simulink model "ThirdCOMController"  (Simulink 7.9)
settings: Solver=ode3  StartTime=0.0  StopTime=inf  RelTol=1e-3
libraries: dspmtrx3 x5, simulink x2, simulink_extras x1, utility x1
settings Model: Creator=jorhabib  LastModifiedBy=jorhabib

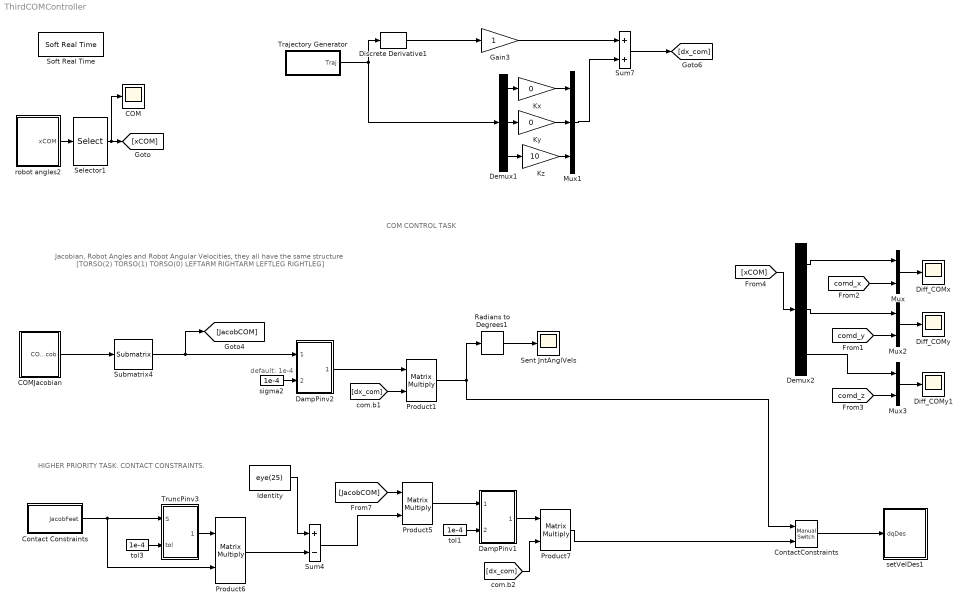
== system ThirdCOMController ==
  note: COM CONTROL TASK
  note: default: 1e-4
  note: Jacobian, Robot Angles and Robot Angular Velocities, they all have the same structure
      | [TORSO(2)  TORSO(1)  TORSO(0)    LEFTARM    RIGHTARM    LEFTLEG    RIGHTLEG]
  note: HIGHER PRIORITY TASK. CONTACT CONSTRAINTS.
  COM : Scope
      settings: TimeRange=100  YMin=-0.1  YMax=0.175
  COMJacobian : Subsystem
  Contact Constraints : Subsystem
  ContactConstraints : simulink/Signal Routing/Manual Switch  sw=1  action=0  varsize=off
  DampPinv1 : Subsystem  mask{tol=1e-4}
      mask prompts: tol "Tolerance"
  DampPinv2 : Subsystem  mask{tol=1e-4}
      mask prompts: tol "Tolerance"
  Demux1 : Demux  Outputs=3
  Demux2 : Demux  Outputs=3
  Diff_COMx : Scope
      settings: TimeRange=100  YMin=0.018  YMax=0.033  SaveName=ScopeData2
  Diff_COMy : Scope
      settings: TimeRange=100  YMin=-0.075  YMax=-0.062  SaveName=ScopeData5
  Diff_COMy1 : Scope
      settings: TimeRange=100  YMin=0.49  YMax=0.55  SaveName=ScopeData3
  Discrete Derivative1 : simulink/Discrete/Discrete Derivative  gainval=1.0  ICPrevScaledInput=0.0  InputProcessing=Inherited  OutMin=[]  OutMax=[]  OutDataType=fixdt(1, 16)  OutScaling=2^-10  DoSatur=off
  Gain3 : Gain
  Identity : Constant  Value=eye(25)
  Kx : Gain  Gain=0
  Ky : Gain  Gain=0
  Kz : Gain  Gain=10
  Mux : Mux  Inputs=2
  Mux1 : Mux  Inputs=3
  Mux2 : Mux  Inputs=2
  Mux3 : Mux  Inputs=2
  Product{1,5..7} (4 alike) : Product  Multiplication=Matrix(*)  RndMeth=Zero
  Radians to Degrees1 : simulink_extras/Transformations/Radians to Degrees
  Selector1 : Selector  IndexMode=Zero-based  InputPortWidth=7  IndexOptions=Index vector (dialog)  Indices=[0:2]  OutputSizes=1
  Sent JntAnglVels : Scope
      settings: YMin=-35  YMax=30  SaveName=ScopeData7
  Soft Real Time : utility/Soft Real Time  x=0.01
  Submatrix4 : dspmtrx3/Submatrix  RowSpan=Range of rows  RowStartMode=First  RowStartIndex=1  RowEndMode=Index  RowEndIndex=3  ColSpan=Range of columns  ColStartMode=Index  ColStartIndex=7  ColEndMode=Last  ColEndIndex=6
  Sum4 : Sum  Inputs=+-
  Sum7 : Sum
  Trajectory Generator : Subsystem
  TruncPinv3 : Subsystem  mask{tol=1e-4}
      mask prompts: tol "Tolerance"
  robot angles2 : Subsystem
  setVelDes1 : Subsystem
  sigma2 : Constant  Value=1e-4
  tol1 : Constant  Value=1e-4
  tol3 : Constant  Value=1e-4
  wires:
  Selector1/1 -> [xCOM], COM/1
  robot angles2/1(xCOM) -> Selector1/1
  Demux1/1 -> Kx/1
  Demux1/2 -> Ky/1
  Kx/1 -> Mux1/1
  Ky/1 -> Mux1/2
  Trajectory Generator/1(Traj) -> Discrete Derivative1/1, Demux1/1
  Mux1/1 -> Sum7/2
  Discrete Derivative1/1 -> Gain3/1
  Gain3/1 -> Sum7/1
  Demux1/3 -> Kz/1
  Kz/1 -> Mux1/3
  sigma2/1 -> DampPinv2/2(sigma)
  Submatrix4/1 -> [JacobCOM], DampPinv2/1(mat)
  DampPinv2/1(DPinv) -> Product1/1
  [dx_com] -> Product1/2
  Product1/1 -> Radians to Degrees1/1, ContactConstraints/1
  Radians to Degrees1/1 -> Sent JntAnglVels/1
  Mux/1 -> Diff_COMx/1
  [comd_x] -> Mux/2
  [comd_y] -> Mux2/2
  Mux2/1 -> Diff_COMy/1
  [xCOM] -> Demux2/1
  Demux2/1 -> Mux/1
  Demux2/2 -> Mux2/1
  COMJacobian/1(COMJacob) -> Submatrix4/1
  [JacobCOM] -> Product5/1
  Identity/1 -> Sum4/1
  tol3/1 -> TruncPinv3/2(tol)
  TruncPinv3/1(Tpinv) -> Product6/1
  Product6/1 -> Sum4/2
  Contact Constraints/1(JacobFeet) -> TruncPinv3/1(S), Product6/2
  Sum4/1 -> Product5/2
  Product5/1 -> DampPinv1/1(mat)
  tol1/1 -> DampPinv1/2(sigma)
  DampPinv1/1(DPinv) -> Product7/1
  [dx_com] -> Product7/2
  Product7/1 -> ContactConstraints/2
  ContactConstraints/1 -> setVelDes1/1(dqDes)
  [comd_z] -> Mux3/2
  Mux3/1 -> Diff_COMy1/1
  Demux2/3 -> Mux3/1
  Sum7/1 -> [dx_com]

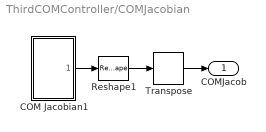
== system ThirdCOMController/COMJacobian ==
  COM Jacobian1 : Subsystem
  Reshape1 : Reshape  OutputDimensionality=Customize  OutputDimensions=[31,6]
  Transpose : dspmtrx3/Transpose  Hermitian=off  overflowFlag=off
  COMJacob : Outport
  wires:
  COM Jacobian1/1(Jacobian) -> Reshape1/1
  Reshape1/1 -> Transpose/1
  Transpose/1 -> COMJacob/1

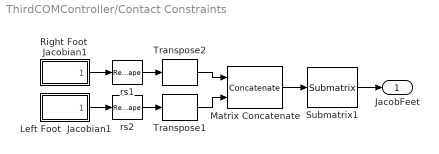
== system ThirdCOMController/Contact Constraints ==
  Left Foot  Jacobian1 : Subsystem
  Matrix Concatenate : Concatenate  Mode=Multidimensional array
  Right Foot  Jacobian1 : Subsystem
  Submatrix1 : dspmtrx3/Submatrix  RowSpan=Range of rows  RowStartMode=First  RowStartIndex=1  RowEndMode=Index  RowEndIndex=3  ColSpan=Range of columns  ColStartMode=Index  ColStartIndex=7  ColEndMode=Last  ColEndIndex=6
  Transpose1 : dspmtrx3/Transpose  Hermitian=off  overflowFlag=off
  Transpose2 : dspmtrx3/Transpose  Hermitian=off  overflowFlag=off
  rs1 : Reshape  OutputDimensionality=Customize  OutputDimensions=[31,6]
  rs2 : Reshape  OutputDimensionality=Customize  OutputDimensions=[31,6]
  JacobFeet : Outport
  wires:
  Right Foot  Jacobian1/1(Jacobian) -> rs1/1
  Left Foot  Jacobian1/1(Jacobian) -> rs2/1
  rs1/1 -> Transpose2/1
  rs2/1 -> Transpose1/1
  Transpose2/1 -> Matrix Concatenate/1
  Transpose1/1 -> Matrix Concatenate/2
  Matrix Concatenate/1 -> Submatrix1/1
  Submatrix1/1 -> JacobFeet/1

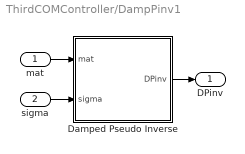
== system ThirdCOMController/DampPinv1 ==
  mat : Inport
  sigma : Inport  Port=2
  Damped Pseudo Inverse : MATLAB Function  TreatAsAtomicUnit=on
  DPinv : Outport
  wires:
  mat/1 -> Damped Pseudo Inverse/1(mat)
  Damped Pseudo Inverse/1(DPinv) -> DPinv/1
  sigma/1 -> Damped Pseudo Inverse/2(sigma)

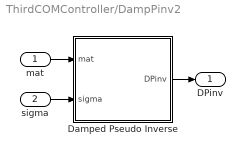
== system ThirdCOMController/DampPinv2 ==
  mat : Inport
  sigma : Inport  Port=2
  Damped Pseudo Inverse : MATLAB Function  TreatAsAtomicUnit=on
  DPinv : Outport
  wires:
  sigma/1 -> Damped Pseudo Inverse/2(sigma)
  Damped Pseudo Inverse/1(DPinv) -> DPinv/1
  mat/1 -> Damped Pseudo Inverse/1(mat)

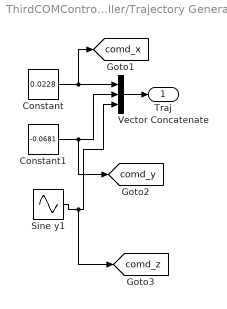
== system ThirdCOMController/Trajectory Generator ==
  Constant : Constant  Value=0.0228  SampleTime=-1
  Constant1 : Constant  Value=-0.0681  SampleTime=-1
  Sine y1 : Sin  Amplitude=0.05  Bias=0.5  Frequency=0.05  Phase=pi
  Vector Concatenate : Concatenate  NumInputs=3
  Traj : Outport
  tag scope: comd_x=global, comd_y=global, comd_z=global
  wires:
  Constant/1 -> Vector Concatenate/1, [comd_x]
  Constant1/1 -> Vector Concatenate/2, [comd_y]
  Vector Concatenate/1 -> Traj/1
  Sine y1/1 -> Vector Concatenate/3, [comd_z]

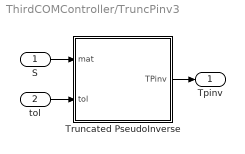
== system ThirdCOMController/TruncPinv3 ==
  S : Inport
  tol : Inport  Port=2
  Truncated PseudoInverse : MATLAB Function  TreatAsAtomicUnit=on
  Tpinv : Outport
  wires:
  tol/1 -> Truncated PseudoInverse/2(tol)
  Truncated PseudoInverse/1(TPinv) -> Tpinv/1
  S/1 -> Truncated PseudoInverse/1(mat)

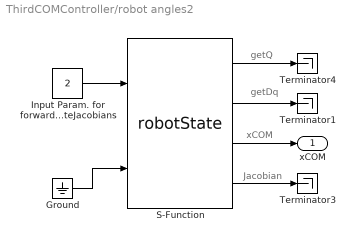
== system ThirdCOMController/robot angles2 ==
  note: getDq
  note: xCOM
  note: getQ
  note: Jacobian
  Ground : Ground
  "Input Param. for forwardKinematics and  computeJacobians " : Constant  Value=2  OutDataTypeStr=int8
  S-Function : S-Function  FunctionName=robotState  Parameters=val,robotname,localname  EnableBusSupport=off  mask{val=2, robotname='icubSim', localname='robotState'}
      mask prompts: val "Value"; robotname "Robot Name (icub - icubSim)"; localname "Module Name"
  Terminator1 : Terminator
  Terminator3 : Terminator
  Terminator4 : Terminator
  xCOM : Outport
  wires:
  Ground/1 -> S-Function/2
  S-Function/2 -> Terminator1/1
  S-Function/1 -> Terminator4/1
  S-Function/3 -> xCOM/1
  "Input Param. for forwardKinematics and  computeJacobians "/1 -> S-Function/1
  S-Function/4 -> Terminator3/1

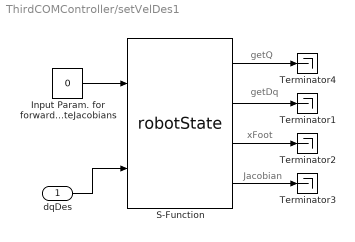
== system ThirdCOMController/setVelDes1 ==
  note: getDq
  note: xFoot
  note: getQ
  note: Jacobian
  dqDes : Inport
  "Input Param. for forwardKinematics and  computeJacobians " : Constant  Value=0  OutDataTypeStr=int8
  S-Function : S-Function  FunctionName=robotState  Parameters=val,robotname,localname  EnableBusSupport=off  mask{val=4, robotname='icubSim', localname='robotState'}
      mask prompts: val "Value"; robotname "Robot Name (icub - icubSim)"; localname "Module Name"
  Terminator{1..4} (4 alike) : Terminator
  wires:
  dqDes/1 -> S-Function/2
  S-Function/2 -> Terminator1/1
  S-Function/1 -> Terminator4/1
  S-Function/3 -> Terminator2/1
  "Input Param. for forwardKinematics and  computeJacobians "/1 -> S-Function/1
  S-Function/4 -> Terminator3/1

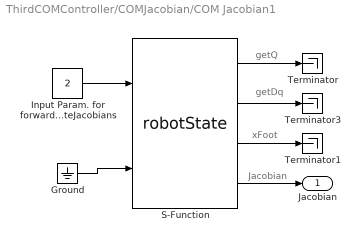
== system ThirdCOMController/COMJacobian/COM Jacobian1 ==
  note: getDq
  note: xFoot
  note: getQ
  note: Jacobian
  Ground : Ground
  "Input Param. for forwardKinematics and  computeJacobians " : Constant  Value=2  OutDataTypeStr=int8
  S-Function : S-Function  FunctionName=robotState  Parameters=val,robotname,localname  EnableBusSupport=off  mask{val=3, robotname='icubSim', localname='robotState'}
      mask prompts: val "Value"; robotname "Robot Name (icub - icubSim)"; localname "Module Name"
  Terminator : Terminator
  Terminator1 : Terminator
  Terminator3 : Terminator
  Jacobian : Outport
  wires:
  Ground/1 -> S-Function/2
  S-Function/2 -> Terminator3/1
  S-Function/1 -> Terminator/1
  S-Function/3 -> Terminator1/1
  "Input Param. for forwardKinematics and  computeJacobians "/1 -> S-Function/1
  S-Function/4 -> Jacobian/1

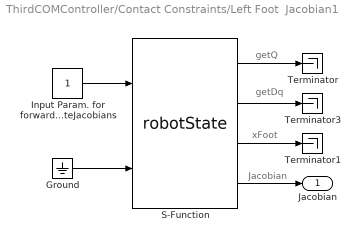
== system ThirdCOMController/Contact Constraints/Left Foot  Jacobian1 ==
  note: Jacobian
  note: getQ
  note: xFoot
  note: getDq
  Ground : Ground
  "Input Param. for forwardKinematics and  computeJacobians " : Constant  OutDataTypeStr=int8
  S-Function : S-Function  FunctionName=robotState  Parameters=val,robotname,localname  EnableBusSupport=off  mask{val=3, robotname='icubSim', localname='robotState'}
      mask prompts: val "Value"; robotname "Robot Name (icub - icubSim)"; localname "Module Name"
  Terminator : Terminator
  Terminator1 : Terminator
  Terminator3 : Terminator
  Jacobian : Outport
  wires:
  S-Function/4 -> Jacobian/1
  "Input Param. for forwardKinematics and  computeJacobians "/1 -> S-Function/1
  S-Function/3 -> Terminator1/1
  S-Function/1 -> Terminator/1
  S-Function/2 -> Terminator3/1
  Ground/1 -> S-Function/2

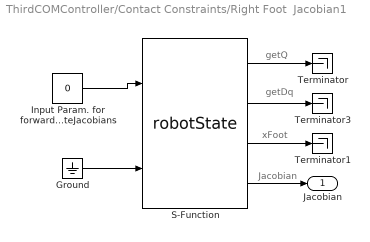
== system ThirdCOMController/Contact Constraints/Right Foot  Jacobian1 ==
  note: getDq
  note: xFoot
  note: getQ
  note: Jacobian
  Ground : Ground
  "Input Param. for forwardKinematics and  computeJacobians " : Constant  Value=0  OutDataTypeStr=int8
  S-Function : S-Function  FunctionName=robotState  Parameters=val,robotname,localname  EnableBusSupport=off  mask{val=3, robotname='icubSim', localname='robotState'}
      mask prompts: val "Value"; robotname "Robot Name (icub - icubSim)"; localname "Module Name"
  Terminator : Terminator
  Terminator1 : Terminator
  Terminator3 : Terminator
  Jacobian : Outport
  wires:
  S-Function/2 -> Terminator3/1
  S-Function/1 -> Terminator/1
  S-Function/3 -> Terminator1/1
  "Input Param. for forwardKinematics and  computeJacobians "/1 -> S-Function/1
  S-Function/4 -> Jacobian/1
  Ground/1 -> S-Function/2

== matlab function DampPinv2/Damped Pseudo Inverse ==
  data: mat input double; DPinv output double; sigma input double
function DPinv  = fcn(mat,sigma)
% Economy size svd of mat
[U,S,V] = svd(mat,'econ');
% Damped version of S with sigma
S(S>sigma)=S(S>sigma)./((S(S>sigma)).^2+sigma^2);
% Damped pseudoinverse
DPinv = V*pinv(S)*U';

== matlab function DampPinv1/Damped Pseudo Inverse ==
  data: mat input double; DPinv output double; sigma input double
function DPinv  = fcn(mat,sigma)
% Economy size svd of mat
[U,S,V] = svd(mat,'econ');
% Damped version of S with sigma
S(S>sigma)=S(S>sigma)./((S(S>sigma)).^2+sigma^2);
% Damped pseudoinverse
DPinv = V*pinv(S)*U';

== matlab function TruncPinv3/Truncated PseudoInverse ==
  data: mat input double; TPinv output double; tol input double
function TPinv  = fcn(mat,tol)
%#codegen
[U,S,V] = svd(mat,'econ');
% Setting to zero value
% Setting to 1/S(i,i) singular values greater than tol
 S(S>tol)=1./S(S>tol);
TPinv = V*pinv(S)*U';
